simulink model "cinematica_inversa_direta"  (R2017b)
settings: Solver=VariableStepAuto  StartTime=0.0  StopTime=5  RelTol=1e-3
settings Model: Creator=jorgeluis  LastModifiedBy=jorgeluis

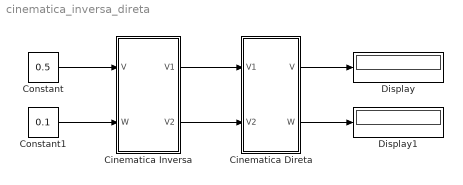
== system cinematica_inversa_direta ==
  Cinematica Direta : Subsystem
  Cinematica Inversa : Subsystem
  Constant : Constant  Value=0.5
  Constant1 : Constant  Value=0.1
  Display : Display
  Display1 : Display
  wires:
  Cinematica Inversa/1(V1) -> Cinematica Direta/1(V1)
  Cinematica Inversa/2(V2) -> Cinematica Direta/2(V2)
  Constant1/1 -> Cinematica Inversa/2(W)
  Constant/1 -> Cinematica Inversa/1(V)
  Cinematica Direta/2(W) -> Display1/1
  Cinematica Direta/1(V) -> Display/1

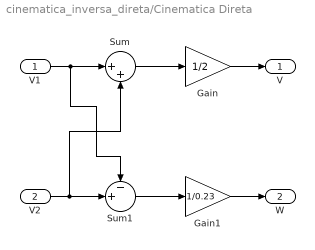
== system cinematica_inversa_direta/Cinematica Direta ==
  V1 : Inport
  V2 : Inport  Port=2
  Gain : Gain  Gain=1/2
  Gain1 : Gain  Gain=1/0.23
  Sum : Sum  Inputs=|++
  Sum1 : Sum  Inputs=-+|
  V : Outport
  W : Outport  Port=2
  wires:
  V2/1 -> Sum/2, Sum1/2
  V1/1 -> Sum1/1, Sum/1
  Sum/1 -> Gain/1
  Gain1/1 -> W/1
  Gain/1 -> V/1
  Sum1/1 -> Gain1/1

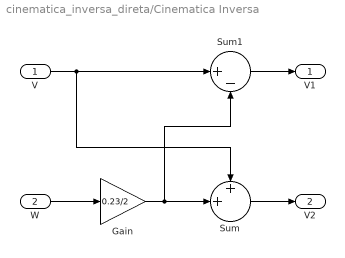
== system cinematica_inversa_direta/Cinematica Inversa ==
  V : Inport
  W : Inport  Port=2
  Gain : Gain  Gain=0.23/2
  Sum : Sum  Inputs=++|
  Sum1 : Sum  Inputs=|+-
  V1 : Outport
  V2 : Outport  Port=2
  wires:
  W/1 -> Gain/1
  Sum1/1 -> V1/1
  Gain/1 -> Sum1/2, Sum/2
  V/1 -> Sum/1, Sum1/1
  Sum/1 -> V2/1
